simulink model "excess3_to_BCD"  (R2025b)
settings: Solver=VariableStepAuto  StartTime=0.0  StopTime=10.0  RelTol=1e-3
settings Model: Creator=jerus  LastModifiedBy=Johan

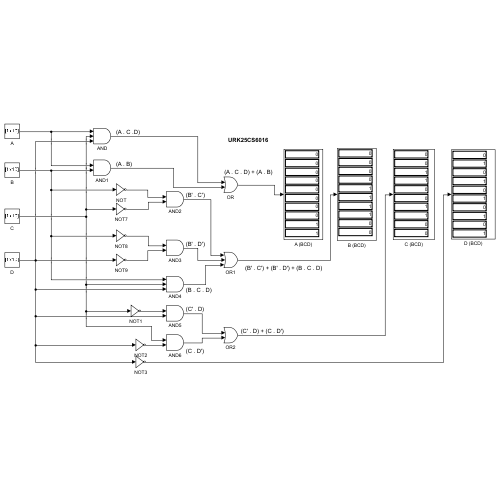
[thumbnail: Simulink's stored preview of the top-level diagram]
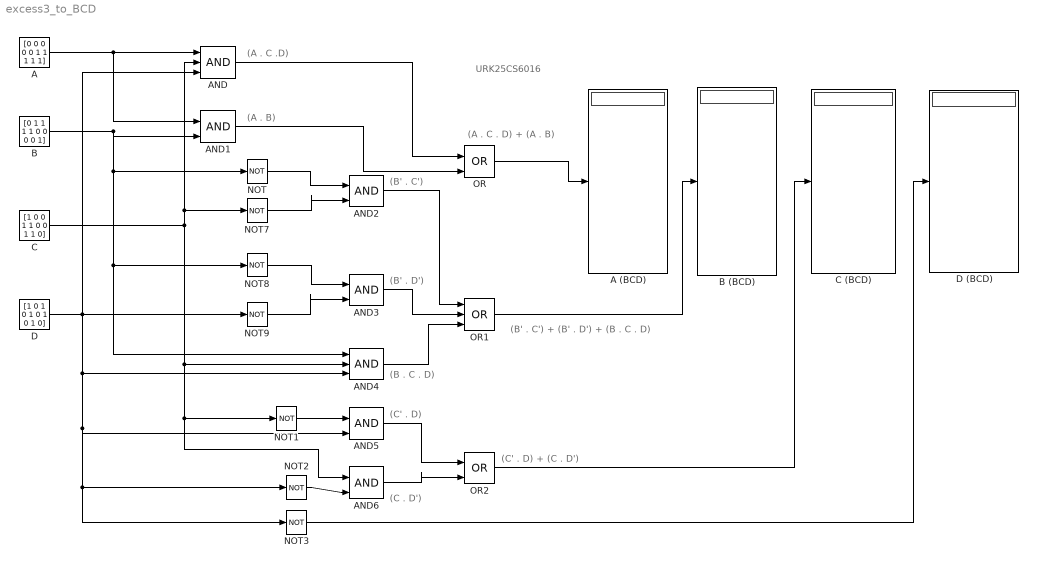
== system excess3_to_BCD ==
  note: (A . C .D)
  note: (A . B)
  note: (A . C . D) + (A . B)
  note: (B' . C')
  note: (B' . D')
  note: (B' . C') + (B' . D') + (B . C . D)
  note: (B . C . D)
  note: (C' . D)
  note: (C . D')
  note: (C' . D) + (C . D')
  note: URK25CS6016
  A : Constant  Value=[0 0 0 0 0 1 1 1 1 1]
  A (BCD) : Display
  AND : Logic  Inputs=3  IconShape=distinctive  AllPortsSameDT=off  OutDataTypeStr=boolean
  AND{1..3,5..6} (5 alike) : Logic  IconShape=distinctive  AllPortsSameDT=off  OutDataTypeStr=boolean
  AND4 : Logic  Inputs=3  IconShape=distinctive  AllPortsSameDT=off  OutDataTypeStr=boolean
  B : Constant  Value=[0 1 1 1 1 0 0 0 0 1]
  B (BCD) : Display
  C : Constant  Value=[1 0 0 1 1 0 0 1 1 0]
  C (BCD) : Display
  D : Constant  Value=[1 0 1 0 1 0 1 0 1 0]
  D (BCD) : Display
  NOT{,1..3,7..9} (7 alike) : Logic  Operator=NOT  IconShape=distinctive  AllPortsSameDT=off  OutDataTypeStr=boolean
  OR : Logic  Operator=OR  IconShape=distinctive  AllPortsSameDT=off  OutDataTypeStr=boolean
  OR1 : Logic  Operator=OR  Inputs=3  IconShape=distinctive  AllPortsSameDT=off  OutDataTypeStr=boolean
  OR2 : Logic  Operator=OR  IconShape=distinctive  AllPortsSameDT=off  OutDataTypeStr=boolean
  wires:
  A/1 -> AND1/1, AND/1
  B/1 -> AND4/1, NOT8/1, NOT/1, AND1/2
  AND/1 -> OR/1
  AND1/1 -> OR/2
  NOT/1 -> AND2/1
  NOT7/1 -> AND2/2
  NOT8/1 -> AND3/1
  NOT9/1 -> AND3/2
  C/1 -> AND/2, NOT7/1, AND6/1, NOT1/1, AND4/2
  D/1 -> NOT9/1, NOT3/1, NOT2/1, AND5/2, AND4/3, AND/3
  NOT1/1 -> AND5/1
  NOT2/1 -> AND6/2
  NOT3/1 -> D (BCD)/1
  AND5/1 -> OR2/1
  AND6/1 -> OR2/2
  AND3/1 -> OR1/2
  AND4/1 -> OR1/3
  OR2/1 -> C (BCD)/1
  OR1/1 -> B (BCD)/1
  OR/1 -> A (BCD)/1
  AND2/1 -> OR1/1
